simulink model "testStateSpace"  (Simulink 7.6)
settings: Solver=ode45  StartTime=0.0  StopTime=0.2  MaxStep=0.01  RelTol=1e-3
settings Model: Creator=guillaume.laurent  LastModifiedBy=guillaume.laurent
settings DebuggingCC: FcnCallInpInsideContextMsg=Enable All  StrictBusMsg=Warning
settings CodeAppCC: CustomSymbolStrType=$N$R$M_T
settings GRTTargetCC: TargetFunctionLibrary=C89/C90 (ANSI)

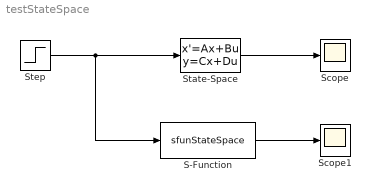
== system testStateSpace ==
  S-Function : S-Function  FunctionName=sfunStateSpace  Parameters="[ -0.09  -0.01 ;  1   ,  0   ]  [  1    -7  ;   0   , -2   ] [  0    2  ;  1   , -5   ] [ -3   0   ;   1   , 0     ]"  SFunctionDeploymentMode=off  EnableBusSupport=off
  Scope : Scope
      settings: TimeRange=auto  LimitDataPoints=on  MaxDataPoints=5000  SaveToWorkspace=off  SaveName=ScopeData  YMin=-4.08633  YMax=2.17885  SampleTime=-1
  Scope1 : Scope
      settings: TimeRange=auto  LimitDataPoints=on  MaxDataPoints=5000  SaveToWorkspace=off  YMin=-0.000000000000000000000000000000000000000000000000000000000000000000000000000000000000000000000000000000000000000000000000000000000000000000000000000000000000000000000000000000000000000000000000000000000000000000000000000000000000000000000000000000000000000000000000000000000000000000000000000000000000000000000000000000000005  YMax=0.000000000000000000000000000000000000000000000000000000000000000000000000000000000000000000000000000000000000000000000000000000000000000000000000000000000000000000000000000000000000000000000000000000000000000000000000000000000000000000000000000000000000000000000000000000000000000000000000000000000000000000000000000000000044  SampleTime=-1
  State-Space : StateSpace  A="[ -0.09  -0.01 ;  1   ,  0   ]"  B="[  1    -7  ;   0   , -2   ]"  C="[  0    2  ;  1   , -5   ]"  D="[ -3   0   ;   1   , 0     ]"  X0=0
  Step : Step  Time=0.1  Before=[0 0]  After=[1 1]  SampleTime=0
  wires:
  Step/1 -> State-Space/1, S-Function/1
  State-Space/1 -> Scope/1
  S-Function/1 -> Scope1/1
